simulink model "exercise2Simu"  (R2020b)
settings: Solver=VariableStepAuto  StartTime=0.0  StopTime=10.0  RelTol=1e-3
values from neighbouring files (symbols this model uses):
  gc = -32.2    [exercise1.m]
  m = mlbm/gc    (= -3.16770186335)    [exercise1.m]
settings Model: Creator=mreiff  LastModifiedBy=mreiff

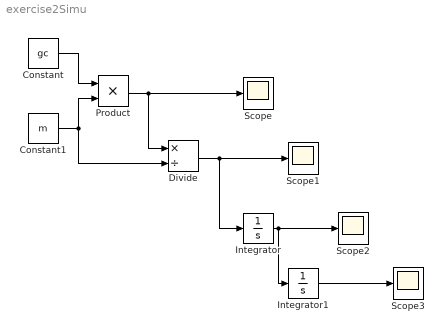
== system exercise2Simu ==
  Constant : Constant  Value=gc
  Constant1 : Constant  Value=m
  Divide : Product  Inputs=*/
  Integrator : Integrator  InitialCondition=200
  Integrator1 : Integrator  InitialCondition=10
  Product : Product
  Scope{,1..3} (4 alike) : Scope
  wires:
  Product/1 -> Divide/1, Scope/1
  Integrator1/1 -> Scope3/1
  Divide/1 -> Scope1/1, Integrator/1
  Integrator/1 -> Integrator1/1, Scope2/1
  Constant1/1 -> Divide/2, Product/2
  Constant/1 -> Product/1
